simulink model "input_system"  (R2018b)
settings: Solver=VariableStepAuto  StartTime=0.0  StopTime=10.0  RelTol=1e-3
undefined symbols (not defined in the file): AM, Am, ffth, frst, frth, O, scnd, t1, t2, t3, t4, thrd, TM, Tm
settings Model: Creator=root  LastModifiedBy=root

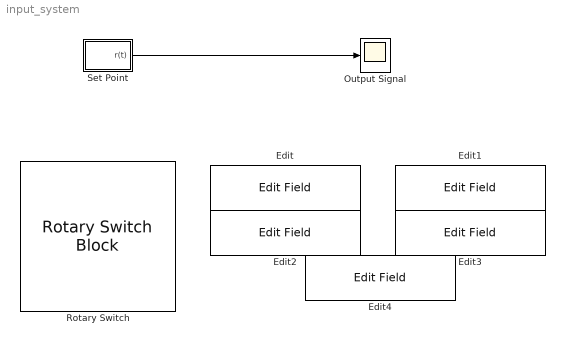
== system input_system ==
  Edit : EditField  WebBlockId=80  ShowInitialText=on  Alignment=Center
  Edit1 : EditField  WebBlockId=81  ShowInitialText=on  Alignment=Center
  Edit2 : EditField  WebBlockId=82  ShowInitialText=on  Alignment=Center
  Edit3 : EditField  WebBlockId=83  ShowInitialText=on  Alignment=Center
  Edit4 : EditField  WebBlockId=84  ShowInitialText=on  Alignment=Center
  Output Signal : Scope
  Rotary Switch : RotarySwitchBlock  WebBlockId=85
      settings: Values={{'Step', 'Sine', 'Sawtooth', 'Square', 'Random'}, [0 1 2 3 4]}
  Set Point : Subsystem
  wires:
  Set Point/1(r(t)) -> Output Signal/1

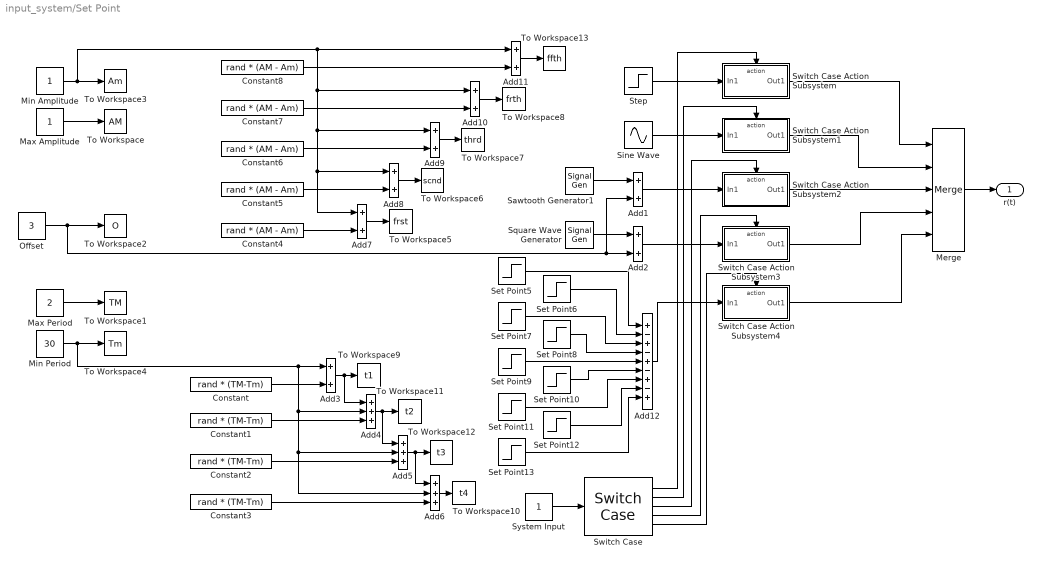
== system input_system/Set Point ==
  Add{1..3,7} (4 alike) : Sum  Inputs=2
  Add{8..11} (4 alike) : Sum
  Add12 : Sum  Inputs=+-+-+-+-+
  Add4 : Sum  Inputs=3
  Add5 : Sum  Inputs=3
  Add6 : Sum  Inputs=3
  Constant{,1..3} (4 alike) : Constant  Value=rand * (TM-Tm)
  Constant{4..8} (5 alike) : Constant  Value=rand * (AM - Am)
  Max Amplitude : Constant  VectorParams1D=off
  Max Period : Constant  Value=2  VectorParams1D=off
  Merge : Merge  Inputs=5
  Min Amplitude : Constant  VectorParams1D=off
  Min Period : Constant  Value=30  VectorParams1D=off
  Offset : Constant  Value=3  VectorParams1D=off
  Sawtooth Generator1 : SignalGenerator  WaveForm=sawtooth  Amplitude=AM  Frequency=1/TM  Units=rad/sec
  Set Point10 : Step  Time=t3  After=thrd  SampleTime=0
  Set Point11 : Step  Time=t3  After=frth  SampleTime=0
  Set Point12 : Step  Time=t4  After=frth  SampleTime=0
  Set Point13 : Step  Time=t4  After=ffth  SampleTime=0
  Set Point5 : Step  Time=0  After=frst  SampleTime=0
  Set Point6 : Step  Time=t1  After=frst  SampleTime=0
  Set Point7 : Step  Time=t1  After=scnd  SampleTime=0
  Set Point8 : Step  Time=t2  After=scnd  SampleTime=0
  Set Point9 : Step  Time=t2  After=thrd  SampleTime=0
  Sine Wave : Sin  Amplitude=AM  Bias=O  Frequency=1/TM  SampleTime=0
  Square Wave Generator : SignalGenerator  WaveForm=square  Amplitude=AM  Frequency=1/TM  Units=rad/sec
  Step : Step  Time=0  After=AM  SampleTime=0
  Switch Case : SwitchCase  CaseConditions={0,1,2,3,4}  ShowDefaultCase=off
  Switch Case Action Subsystem : Subsystem  TreatAsAtomicUnit=on
  Switch Case Action Subsystem1 : Subsystem  TreatAsAtomicUnit=on
  Switch Case Action Subsystem2 : Subsystem  TreatAsAtomicUnit=on
  Switch Case Action Subsystem3 : Subsystem  TreatAsAtomicUnit=on
  Switch Case Action Subsystem4 : Subsystem  TreatAsAtomicUnit=on
  System Input : Constant
  To Workspace : ToWorkspace  VariableName=AM  SampleTime=-1
      settings: MaxDataPoints=1
  To Workspace1 : ToWorkspace  VariableName=TM  SampleTime=-1
      settings: MaxDataPoints=1
  To Workspace10 : ToWorkspace  VariableName=t4  SampleTime=-1
      settings: MaxDataPoints=1
  To Workspace11 : ToWorkspace  VariableName=t2  SampleTime=-1
      settings: MaxDataPoints=1
  To Workspace12 : ToWorkspace  VariableName=t3  SampleTime=-1
      settings: MaxDataPoints=1
  To Workspace13 : ToWorkspace  VariableName=ffth  SampleTime=-1
      settings: MaxDataPoints=1
  To Workspace2 : ToWorkspace  VariableName=O  SampleTime=-1
      settings: MaxDataPoints=1
  To Workspace3 : ToWorkspace  VariableName=Am  SampleTime=-1
      settings: MaxDataPoints=1
  To Workspace4 : ToWorkspace  VariableName=Tm  SampleTime=-1
      settings: MaxDataPoints=1
  To Workspace5 : ToWorkspace  VariableName=frst  SampleTime=-1
      settings: MaxDataPoints=1
  To Workspace6 : ToWorkspace  VariableName=scnd  SampleTime=-1
      settings: MaxDataPoints=1
  To Workspace7 : ToWorkspace  VariableName=thrd  SampleTime=-1
      settings: MaxDataPoints=1
  To Workspace8 : ToWorkspace  VariableName=frth  SampleTime=-1
      settings: MaxDataPoints=1
  To Workspace9 : ToWorkspace  VariableName=t1  SampleTime=-1
      settings: MaxDataPoints=1
  r(t) : Outport
  wires:
  Merge/1 -> r(t)/1
  Switch Case Action Subsystem3/1(Out1) -> Merge/4
  Switch Case/1 -> Switch Case Action Subsystem/Action
  Max Amplitude/1 -> To Workspace/1
  Square Wave Generator/1 -> Add2/1
  Add1/1 -> Switch Case Action Subsystem2/1(In1)
  Step/1 -> Switch Case Action Subsystem/1(In1)
  Switch Case/3 -> Switch Case Action Subsystem2/Action
  Switch Case/4 -> Switch Case Action Subsystem3/Action
  Switch Case/5 -> Switch Case Action Subsystem4/Action
  Switch Case/2 -> Switch Case Action Subsystem1/Action
  Sawtooth Generator1/1 -> Add1/1
  System Input/1 -> Switch Case/1
  Switch Case Action Subsystem/1(Out1) -> Merge/1
  Add2/1 -> Switch Case Action Subsystem3/1(In1)
  Min Amplitude/1 -> To Workspace3/1, Add7/1, Add8/1, Add9/1, Add10/1, Add11/1
  Max Period/1 -> To Workspace1/1
  Offset/1 -> Add1/2, Add2/2, To Workspace2/1
  Switch Case Action Subsystem4/1(Out1) -> Merge/5
  Switch Case Action Subsystem2/1(Out1) -> Merge/3
  Sine Wave/1 -> Switch Case Action Subsystem1/1(In1)
  Switch Case Action Subsystem1/1(Out1) -> Merge/2
  Min Period/1 -> To Workspace4/1, Add6/2, Add5/2, Add4/2, Add3/1
  Add12/1 -> Switch Case Action Subsystem4/1(In1)
  Constant/1 -> Add3/2
  Add3/1 -> Add4/1, To Workspace9/1
  Add4/1 -> Add5/1, To Workspace11/1
  Constant1/1 -> Add4/3
  Constant2/1 -> Add5/3
  Add6/1 -> To Workspace10/1
  Add5/1 -> Add6/1, To Workspace12/1
  Constant3/1 -> Add6/3
  Add8/1 -> To Workspace6/1
  Add10/1 -> To Workspace8/1
  Add9/1 -> To Workspace7/1
  Add7/1 -> To Workspace5/1
  Constant4/1 -> Add7/2
  Constant5/1 -> Add8/2
  Constant6/1 -> Add9/2
  Constant7/1 -> Add10/2
  Add11/1 -> To Workspace13/1
  Constant8/1 -> Add11/2
  Set Point13/1 -> Add12/9
  Set Point11/1 -> Add12/7
  Set Point9/1 -> Add12/5
  Set Point8/1 -> Add12/4
  Set Point5/1 -> Add12/1
  Set Point12/1 -> Add12/8
  Set Point7/1 -> Add12/3
  Set Point10/1 -> Add12/6
  Set Point6/1 -> Add12/2

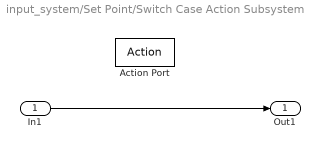
== system input_system/Set Point/Switch Case Action Subsystem ==
  In1 : Inport
  Action Port : ActionPort  ActionType=case
  Out1 : Outport
  wires:
  In1/1 -> Out1/1

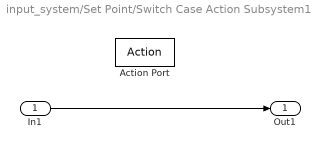
== system input_system/Set Point/Switch Case Action Subsystem1 ==
  In1 : Inport
  Action Port : ActionPort  ActionType=case
  Out1 : Outport
  wires:
  In1/1 -> Out1/1

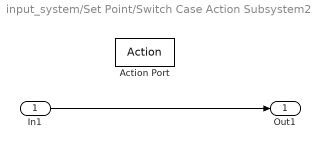
== system input_system/Set Point/Switch Case Action Subsystem2 ==
  In1 : Inport
  Action Port : ActionPort  ActionType=case
  Out1 : Outport
  wires:
  In1/1 -> Out1/1

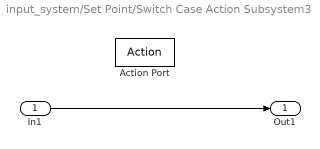
== system input_system/Set Point/Switch Case Action Subsystem3 ==
  In1 : Inport
  Action Port : ActionPort  ActionType=case
  Out1 : Outport
  wires:
  In1/1 -> Out1/1

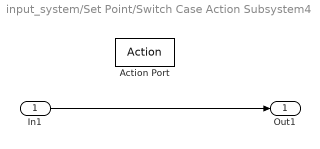
== system input_system/Set Point/Switch Case Action Subsystem4 ==
  In1 : Inport
  Action Port : ActionPort  ActionType=case
  Out1 : Outport
  wires:
  In1/1 -> Out1/1
